simulink model "p1a"  (R2017b)
settings: Solver=FixedStepAuto  StartTime=0.0  StopTime=10.0  FixedStep=0.01  RelTol=1e-3
undefined symbols (not defined in the file): a, b, c, K
settings Model: Creator=Soutrik  LastModifiedBy=Soutrik

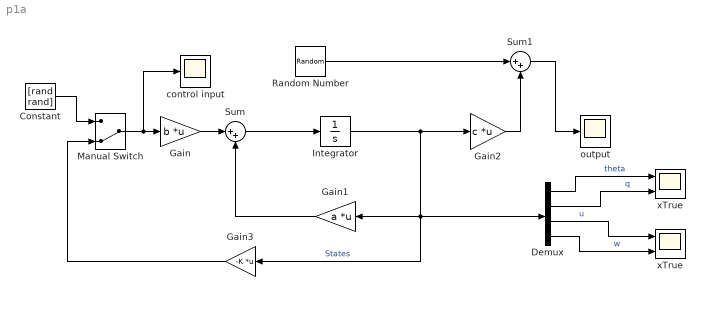
== system p1a ==
  Constant : Constant  Value=[rand rand]
  Demux : Demux
  Gain : Gain  Gain=b  Multiplication=Matrix(K*u)
  Gain1 : Gain  Gain=a  Multiplication=Matrix(K*u)
  Gain2 : Gain  Gain=c  Multiplication=Matrix(K*u)
  Gain3 : Gain  Gain=-K  Multiplication=Matrix(K*u)
  Integrator : Integrator  InitialCondition=[0.05 0 0 0]
  Manual Switch : ManualSwitch  CurrentSetting=0
  Random Number : RandomNumber  Variance=[0.00001, 0.00001, 0.0001, 0.0001]  Seed=[1 2 3 4]  SampleTime=0.01
  Sum : Sum  Inputs=|++
  Sum1 : Sum  Inputs=|++
  control input : Scope
  output : Scope
  xTrue : Scope  NumInputPorts=2
  "xTrue " : Scope  NumInputPorts=2
  wires:
  Sum/1 -> Integrator/1
  Constant/1 -> Manual Switch/1
  Demux/4 -> "xTrue "/2  "w"
  Demux/1 -> xTrue/1  "theta"
  Demux/2 -> xTrue/2  "q"
  Gain/1 -> Sum/1
  Integrator/1 -> Gain3/1, Demux/1, Gain1/1, Gain2/1  "States"
  Gain3/1 -> Manual Switch/2
  Demux/3 -> "xTrue "/1  "u"
  Gain1/1 -> Sum/2
  Manual Switch/1 -> control input/1, Gain/1
  Random Number/1 -> Sum1/1
  Gain2/1 -> Sum1/2
  Sum1/1 -> output/1
